simulink model "reichardt_array_EMD_3"  (R2018b)
settings: Solver=ode45  StartTime=0.0  StopTime=setStopTime  FixedStep=0.0005  RelTol=1e-3  EnableMultiTasking=on
model workspace (MAT data in the model file):
  bodyAmp = 0
  bodyPhase = 0
  freq = 0.832969017384
  headAmp = 0
  headPhase = 0
  imageData = [0.00228480667088 0.00685422825671 0.0114230745906 0.0159909622235 0.0205575077854 0.0251223280162 0.0296850397975 0.0342452601838 0.0388026064343 0.0433566960441 0.0479071467754 0.0524535766893 ... (8204 elements, 1x8204)]
  outputTimeList = [7.54312006335 7.61855126399 7.69398246462 7.76941366526 7.84484486589 7.92027606652 7.99570726716 8.07113846779 8.14656966842 8.22200086906 8.29743206969 8.37286327032 8.44829447096 8.52372567159 8.59915687222 8.67458807286 8.75001927349 8.82545047412 8.90088167476 8.97631287539 9.05174407603 9.12717527666 9.20260647729 9.27803767793 9.35346887856 9.42890007919 9.50433127983 9.57976248046 9.65519368109 9.73062488173 9.80605608236 9.88148728299 9.95691848363 10.0323496843 10.1077808849 10.1832120855 10.2586432862 10.3340744868 10.4095056874 10.4849368881 10.5603680887 10.6357992893 10.71123049 10.7866616906 10.8620928912 10.9375240919 11.0129552925 11.0883864931 11.1638176938 11.2392488944 11.314680095 11.3901112957 11.4655424963 11.5409736969 11.6164048976 11.6918360982 11.7672672988 11.8426984995 11.9181297001 11.9935609007 12.0689921014 12.144423302 12.2198545026 12.2952857033 12.3707169039 12.4461481045 12.5215793052 12.5970105058 12.6724417064 12.7478729071 12.8233041077 12.8987353083 12.974166509 13.0495977096 13.1250289102 13.2004601109 13.2758913115 13.3513225121 13.4267537128 13.5021849134 13.577616114 13.6530473147 13.7284785153 13.8039097159 13.8793409166 13.9547721172 14.0302033178 14.1056345185 14.1810657191 14.2564969197 14.3319281204 14.407359321 14.4827905216 14.5582217223 14.6336529229 14.7090841235 14.7845153242 14.8599465248 14.9353777254 15.0108089261 15.0862401267]
  setStopTime = 15.0862401267
  stimAmp = 15
  temporalFilt = 0.035
  timeConstant = 0.035
libraries: visionsources x1
(part 1 of 2)
settings Model: SimulationMode=accelerator  Creator=Shane  LastModifiedBy=boc5244
settings DataIOCC: SaveFormat=Array  ReturnWorkspaceOutputs=on  OutputOption=SpecifiedOutputTimes  OutputTimes=outputTimeList
settings OptimizationCC: ExpressionDepthLimit=2147483647  EfficientMapNaN2IntZero=off  SimCompilerOptimization=on
settings DebuggingCC: UnderspecifiedInitializationDetection=Classic  MergeDetectMultiDrivingBlocksExec=none  FcnCallInpInsideContextMsg=warning  StateNameClashWarn=warning  SFUnexpectedBacktrackingDiag=warning  SFNoUnconditionalDefaultTransitionDiag=warning  SFExecutionAtInitializationDiag=none
settings HardwareCC: ProdBitPerPointer=32  ProdBitPerSizeT=32  ProdBitPerPtrDiffT=32  ProdLargestAtomicFloat=None  ProdIntDivRoundTo=Undefined  ProdEndianess=Unspecified  ProdWordSize=32  ProdHWDeviceType=32-bit Generic  TargetBitPerPointer=64  TargetBitPerSizeT=64  TargetBitPerPtrDiffT=64  TargetLongLongMode=on  TargetIntDivRoundTo=Zero  TargetEndianess=LittleEndian  TargetWordSize=64  TargetHWDeviceType=MATLAB Host  ProdEqTarget=off
settings ModelReferenceCC: PropagateSignalLabelsOutOfModel=off
settings SFSimCC: SimUseLocalCustomCode=off
settings RTWCC: SystemTargetFile=accel.tlc  TemplateMakefile=accel_default_tmf  RTWVerbose=off
settings CodeAppCC: MaxIdLength=128
settings STFCustomTargetCC: ConcurrentExecutionCompliant=on  MATLABClassNameForMDSCustomization=Simulink.SoftwareTarget.TargetSpecificTriggerConfigurationBase  GRTInterface=on  SystemTargetFile=accel.tlc
settings ConfigComp: CovMetricSettings=dw  CovHtmlReporting=on  CovSaveCumulativeToWorkspaceVar=on  CovSaveSingleToWorkspaceVar=on  CovExternalEMLEnable=off

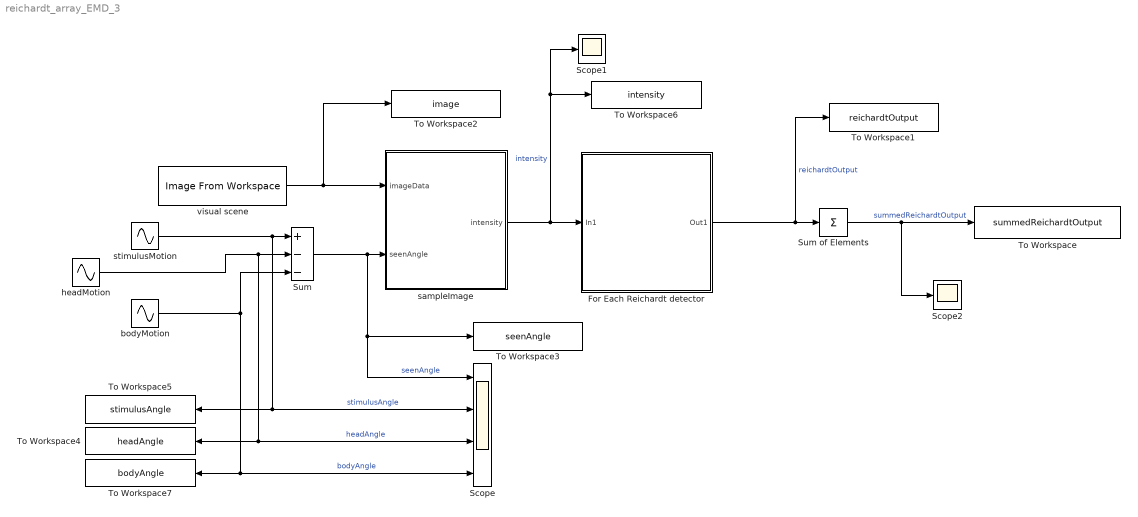
== system reichardt_array_EMD_3 ==
  For Each Reichardt detector : Subsystem  TreatAsAtomicUnit=on
  Scope : Scope  NumInputPorts=4
  Scope1 : Scope
  Scope2 : Scope
  Sum : Sum  Inputs=+--
  Sum of Elements : Sum  Inputs=+
  To Workspace : ToWorkspace  VariableName=summedReichardtOutput  SaveFormat=Timeseries  SampleTime=-1
  To Workspace1 : ToWorkspace  VariableName=reichardtOutput  SaveFormat=Timeseries  SampleTime=-1
  To Workspace2 : ToWorkspace  VariableName=image  SaveFormat=Timeseries  SampleTime=-1
  To Workspace3 : ToWorkspace  VariableName=seenAngle  SaveFormat=Timeseries  SampleTime=-1
  To Workspace4 : ToWorkspace  VariableName=headAngle  SaveFormat=Timeseries  SampleTime=-1
  To Workspace5 : ToWorkspace  VariableName=stimulusAngle  SaveFormat=Timeseries  SampleTime=-1
  To Workspace6 : ToWorkspace  VariableName=intensity  SaveFormat=Timeseries  SampleTime=-1
  To Workspace7 : ToWorkspace  VariableName=bodyAngle  SaveFormat=Timeseries  SampleTime=-1
  bodyMotion : Sin  Amplitude=bodyAmp  Frequency=freq  Phase=bodyPhase  SampleTime=0
  headMotion : Sin  Amplitude=headAmp  Frequency=freq  Phase=headPhase  SampleTime=0
  sampleImage : MATLAB Function  TreatAsAtomicUnit=on
  stimulusMotion : Sin  Amplitude=stimAmp  Frequency=freq  SampleTime=0
  visual scene : visionsources/Image From Workspace  Tag=vipblks_nd  ImageValue=imageData  Ts=inf  imagePorts=One multidimensional signal  OutPortLabels=R|G|B  ImageDataType=double  Signed=on  WordLength=16  sdImageDataType=sfix(16)  FractionLengthMode=User-defined  FractionLength=15
      settings: SourceProductName=Computer Vision Toolbox  SourceProductBaseCode=VP
  wires:
  For Each Reichardt detector/1(Out1) -> To Workspace1/1, Sum of Elements/1  "reichardtOutput"
  Sum of Elements/1 -> Scope2/1, To Workspace/1  "summedReichardtOutput"
  sampleImage/1(intensity) -> Scope1/1, To Workspace6/1, For Each Reichardt detector/1(In1)  "intensity"
  visual scene/1 -> To Workspace2/1, sampleImage/1(imageData)
  stimulusMotion/1 -> To Workspace5/1, Scope/2, Sum/1  "stimulusAngle"
  headMotion/1 -> To Workspace4/1, Scope/3, Sum/2  "headAngle"
  Sum/1 -> Scope/1, To Workspace3/1, sampleImage/2(seenAngle)  "seenAngle"
  bodyMotion/1 -> Sum/3, To Workspace7/1, Scope/4  "bodyAngle"
